simulink model "lab2_floatp"  (R2022a)
settings: Solver=VariableStepAuto  StartTime=0.0  StopTime=10.0  RelTol=1e-3
settings Model: Creator=user  LastModifiedBy=user

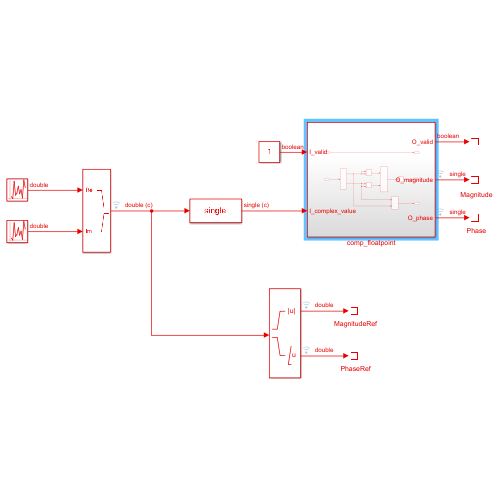
[thumbnail: Simulink's stored preview of the top-level diagram]
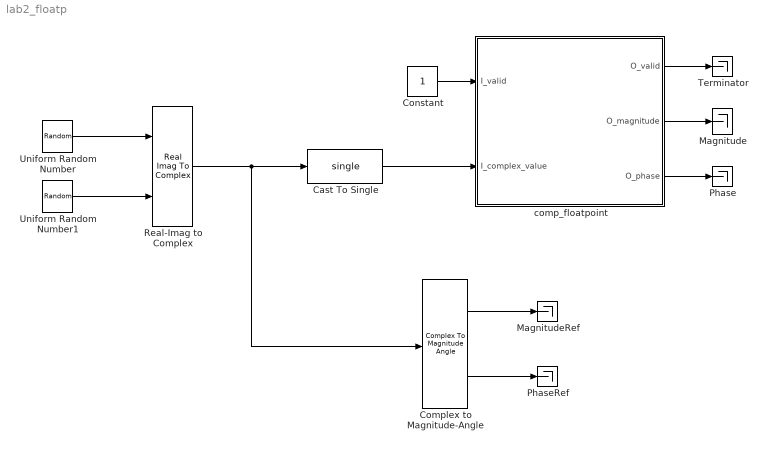
== system lab2_floatp ==
  Cast To Single : DataTypeConversion  OutDataTypeStr=single  SaturateOnIntegerOverflow=off  RndMeth=Floor
  Complex to Magnitude-Angle : ComplexToMagnitudeAngle
  Constant : Constant  OutDataTypeStr=boolean  SampleTime=1
  Magnitude : Terminator
  MagnitudeRef : Terminator
  Phase : Terminator
  PhaseRef : Terminator
  Real-Imag to Complex : RealImagToComplex
  Terminator : Terminator
  Uniform Random Number : UniformRandomNumber  Minimum=0  Maximum=1023.99999976158142089844  Seed=10  SampleTime=1
  Uniform Random Number1 : UniformRandomNumber  Minimum=0  Maximum=1023.999999761581420898441  Seed=11  SampleTime=1
  comp_floatpoint : Subsystem
  wires:
  Uniform Random Number1/1 -> Real-Imag to Complex/2
  Uniform Random Number/1 -> Real-Imag to Complex/1
  Real-Imag to Complex/1 -> Cast To Single/1, Complex to Magnitude-Angle/1
  Constant/1 -> comp_floatpoint/1(I_valid)
  comp_floatpoint/1(O_valid) -> Terminator/1
  Cast To Single/1 -> comp_floatpoint/2(I_complex_value)
  comp_floatpoint/3(O_phase) -> Phase/1
  comp_floatpoint/2(O_magnitude) -> Magnitude/1
  Complex to Magnitude-Angle/1 -> MagnitudeRef/1
  Complex to Magnitude-Angle/2 -> PhaseRef/1

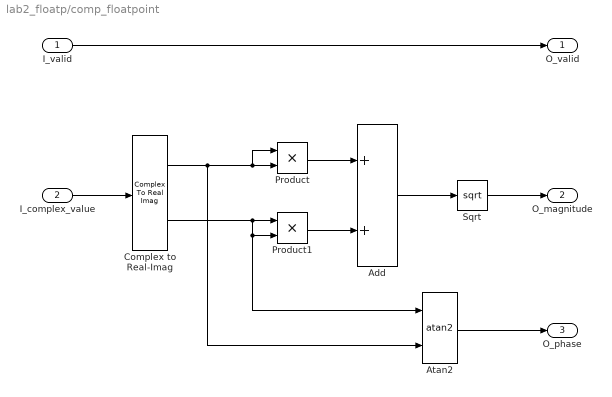
== system lab2_floatp/comp_floatpoint ==
  I_valid : Inport
  I_complex_value : Inport  Port=2
  Add : Sum
  Atan2 : Trigonometry  Operator=atan2
  Complex to Real-Imag : ComplexToRealImag
  Product : Product
  Product1 : Product
  Sqrt : Sqrt
  O_valid : Outport
  O_magnitude : Outport  Port=2
  O_phase : Outport  Port=3
  wires:
  I_valid/1 -> O_valid/1
  I_complex_value/1 -> Complex to Real-Imag/1
  Complex to Real-Imag/1 -> Atan2/2, Product/1, Product/2
  Complex to Real-Imag/2 -> Atan2/1, Product1/2, Product1/1
  Product1/1 -> Add/2
  Product/1 -> Add/1
  Add/1 -> Sqrt/1
  Sqrt/1 -> O_magnitude/1
  Atan2/1 -> O_phase/1
